simulink model "lqr_terrain_following"  (R2018b)
settings: Solver=VariableStepAuto  StartTime=0.0  StopTime=60  RelTol=1e-3
values from neighbouring files (symbols this model uses):
  A_red = aircraft_long.A([2, 4], [2, 4])    [reduced_2_state_model.m]    (also in terrain_following_model.m = A([3, 7, 8, 5, 11], [3, 7, 8, 5 11]))
  B_red = aircraft_long.B([2, 4])    [reduced_2_state_model.m]    (also in terrain_following_model.m = A([3, 7, 8, 5, 11], [13, 14]))
  C_red = aircraft_long.C([2, 4], [2, 4])    [reduced_2_state_model.m]    (also in terrain_following_model.m = eye(5))
  D_red = 0    [reduced_2_state_model.m]    (also in terrain_following_model.m = D([3, 7, 8, 5, 11], [1, 2]))
  K_h = K(:, 1)    [terrain_following_model.m]
  K_inner = K(:, 2:end)    [terrain_following_model.m]
  trim_state_lin = trim_state_lo    [FindF16Dynamics.m]    (also in runLINF16sim.m; terrain_following_model.m = [trim.trim_state_lo; trim.trim_thrust_lo; trim.trim_control_)
settings Model: Creator=lorenzoterenzi  LastModifiedBy=lorenzoterenzi

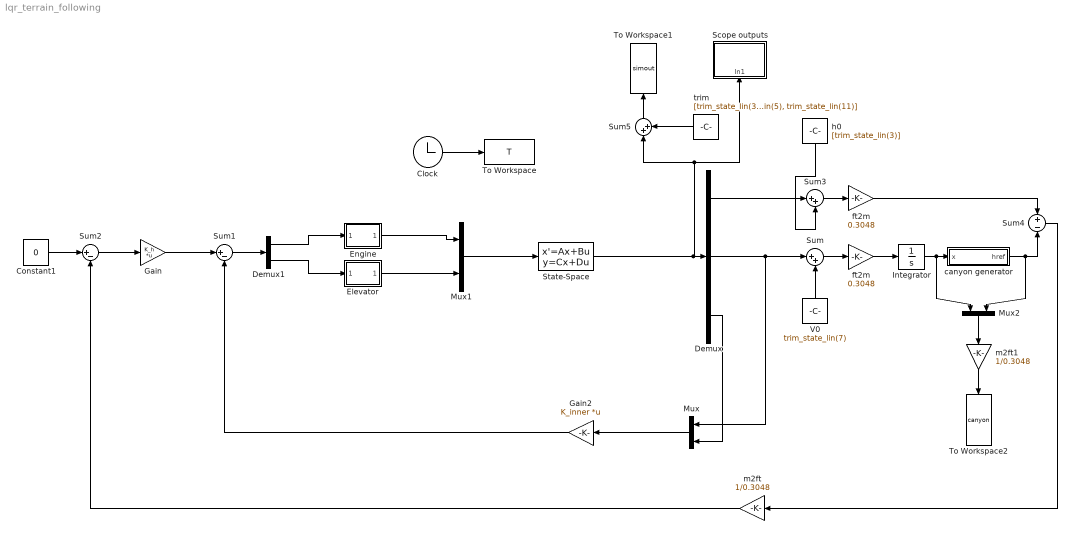
== system lqr_terrain_following ==
  Clock : Clock
      settings: Decimation=50
  Constant1 : Constant  Value=0
  Demux : Demux  Outputs=[1 1 3]
  Demux1 : Demux  Outputs=2
  Elevator : Subsystem
  Engine : Subsystem
  Gain : Gain  Gain=K_h  Multiplication=Matrix(K*u)
  Gain2 : Gain  Gain=K_inner  Multiplication=Matrix(K*u)
  Integrator : Integrator
  Mux : Mux  Inputs=2
  Mux1 : Mux  Inputs=2
  Mux2 : Mux  Inputs=2
  Scope outputs : Subsystem
  State-Space : StateSpace  A=A_red  B=B_red  C=C_red  D=D_red  InitialCondition=[1500/0.3048 - 5000, 0, 0, 0, 0]
  Sum : Sum  Inputs=|++
  Sum1 : Sum  Inputs=|+-
  Sum2 : Sum  Inputs=|+-
  Sum3 : Sum  Inputs=|++
  Sum4 : Sum  Inputs=+|-
  Sum5 : Sum  Inputs=|++
  To Workspace : ToWorkspace  VariableName=T  SampleTime=-1
      settings: Decimation=100
  To Workspace1 : ToWorkspace  VariableName=simout  SaveFormat=Timeseries  SampleTime=-1
  To Workspace2 : ToWorkspace  VariableName=canyon  SaveFormat=Timeseries  SampleTime=-1
  V0 : Constant  Value=trim_state_lin(7)
  canyon generator : Subsystem
      mask Display: image(imread('refalt.jpg'))
  ft2m : Gain  Gain=0.3048
  "ft2m " : Gain  Gain=0.3048
  "h0 " : Constant  Value=[trim_state_lin(3)]
  m2ft : Gain  Gain=1/0.3048
  m2ft1 : Gain  Gain=1/0.3048
  trim : Constant  Value=[trim_state_lin(3), trim_state_lin(7), trim_state_lin(8), trim_state_lin(5), trim_state_lin(11)]
  wires:
  Mux1/1 -> State-Space/1
  Engine/1(Out1) -> Mux1/1
  Elevator/1(Out1) -> Mux1/2
  State-Space/1 -> Sum5/1, Scope outputs/1(In1), Demux/1
  Clock/1 -> To Workspace/1
  Integrator/1 -> Mux2/1, canyon generator/1(x)
  Sum4/1 -> m2ft/1
  Constant1/1 -> Sum2/1
  Demux/2 -> Sum/1, Mux/1
  Demux/3 -> Mux/2
  Mux/1 -> Gain2/1
  Gain2/1 -> Sum1/2
  Demux1/1 -> Engine/1(In1)
  Demux1/2 -> Elevator/1(In1)
  Sum/1 -> "ft2m "/1
  V0/1 -> Sum/2
  "ft2m "/1 -> Integrator/1
  Demux/1 -> Sum3/1
  "h0 "/1 -> Sum3/2
  Sum3/1 -> ft2m/1
  ft2m/1 -> Sum4/1
  Sum2/1 -> Gain/1
  Gain/1 -> Sum1/1
  Sum1/1 -> Demux1/1
  m2ft/1 -> Sum2/2
  trim/1 -> Sum5/2
  Sum5/1 -> To Workspace1/1
  canyon generator/1(href) -> Mux2/2, Sum4/2
  Mux2/1 -> m2ft1/1
  m2ft1/1 -> To Workspace2/1

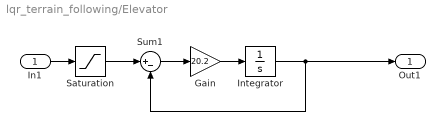
== system lqr_terrain_following/Elevator ==
  In1 : Inport
  Gain : Gain  Gain=20.2
  Integrator : Integrator
  Saturation : Saturate  UpperLimit=25 - trim_state_lin(14)  LowerLimit=-25 - trim_state_lin(14)
  Sum1 : Sum  Inputs=|+-
  Out1 : Outport
  wires:
  Gain/1 -> Integrator/1
  Sum1/1 -> Gain/1
  Integrator/1 -> Out1/1, Sum1/2
  In1/1 -> Saturation/1
  Saturation/1 -> Sum1/1

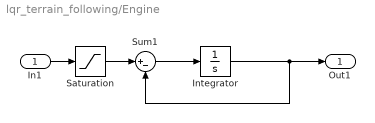
== system lqr_terrain_following/Engine ==
  In1 : Inport
  Integrator : Integrator
  Saturation : Saturate  UpperLimit=19000 - trim_state_lin(13)  LowerLimit=1000 - trim_state_lin(13)
  Sum1 : Sum  Inputs=|+-
  Out1 : Outport
  wires:
  Sum1/1 -> Integrator/1
  Integrator/1 -> Sum1/2, Out1/1
  In1/1 -> Saturation/1
  Saturation/1 -> Sum1/1

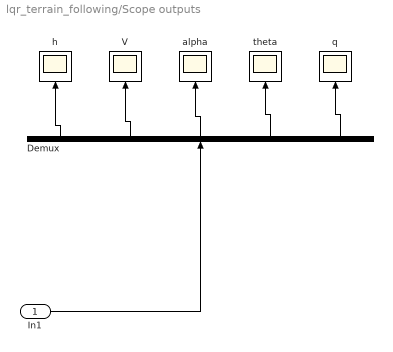
== system lqr_terrain_following/Scope outputs ==
  In1 : Inport
  Demux : Demux  Outputs=5
  V : Scope
  alpha : Scope
  h : Scope
  q : Scope
  theta : Scope
  wires:
  In1/1 -> Demux/1
  Demux/1 -> h/1
  Demux/3 -> alpha/1
  Demux/2 -> V/1
  Demux/5 -> q/1
  Demux/4 -> theta/1

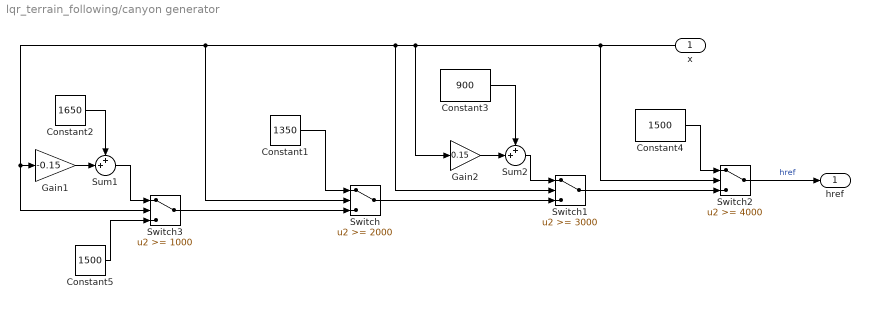
== system lqr_terrain_following/canyon generator ==
  x : Inport
  Constant1 : Constant  Value=1350
  Constant2 : Constant  Value=1650
  Constant3 : Constant  Value=900
  Constant4 : Constant  Value=1500
  Constant5 : Constant  Value=1500
  Gain1 : Gain  Gain=-0.15
  Gain2 : Gain  Gain=0.15
  Sum1 : Sum  Inputs=++|
  Sum2 : Sum  Inputs=++|
  Switch : Switch  Threshold=2000  ZeroCross=off
  Switch1 : Switch  Threshold=3000  ZeroCross=off
  Switch2 : Switch  Threshold=4000  ZeroCross=off
  Switch3 : Switch  Threshold=1000  ZeroCross=off
  href : Outport
  wires:
  Constant1/1 -> Switch/1
  x/1 -> Switch2/2, Gain2/1, Switch1/2, Switch/2, Gain1/1, Switch3/2
  Switch/1 -> Switch1/3
  Gain2/1 -> Sum2/2
  Constant3/1 -> Sum2/1
  Sum2/1 -> Switch1/1
  Switch1/1 -> Switch2/3
  Constant4/1 -> Switch2/1
  Switch2/1 -> href/1  "href"
  Switch3/1 -> Switch/3
  Constant5/1 -> Switch3/3
  Sum1/1 -> Switch3/1
  Gain1/1 -> Sum1/2
  Constant2/1 -> Sum1/1
